simulink model "Registro_Harness2"  (R2020a)
settings: Solver=VariableStepAuto  StartTime=0.0  StopTime=10.0  RelTol=1e-3
settings Model: DataDictionary=Registro_variables.sldd  Creator=Juan  LastModifiedBy=Juan

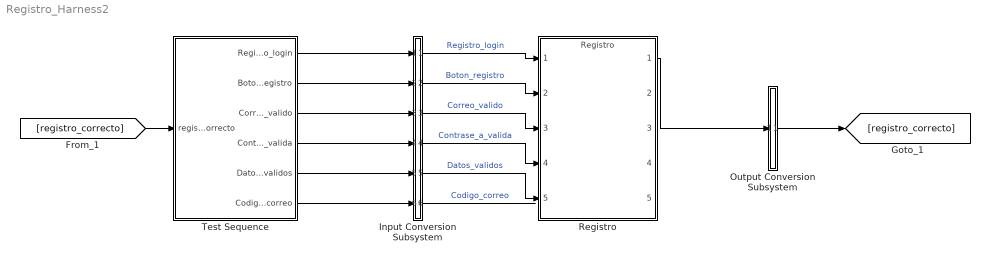
== system Registro_Harness2 ==
  Input Conversion Subsystem : Subsystem  Tag=__SLT_ICS__  Description=|
      | Signal spec.
      | and routing
      settings: AttributesFormatString=%<Description>
  Output Conversion Subsystem : Subsystem  Tag=__SLT_OCS__  Description=|
      | Signal spec.
      | and routing
      settings: AttributesFormatString=%<Description>
  Registro : ModelReference  ModelNameDialog=Registro  SimulationMode=Normal  ModelReferenceVersion=1.29
  Test Sequence : Test Sequence  TreatAsAtomicUnit=on
  wires:
  Test Sequence/1(Registro_login) -> Input Conversion Subsystem/1(Inport_1)
  Test Sequence/2(Boton_registro) -> Input Conversion Subsystem/2(Inport_2)
  Test Sequence/3(Correo_valido) -> Input Conversion Subsystem/3(Inport_3)
  Test Sequence/4(Contrase_a_valida) -> Input Conversion Subsystem/4(Inport_4)
  Test Sequence/5(Datos_validos) -> Input Conversion Subsystem/5(Inport_5)
  Test Sequence/6(Codigo_correo) -> Input Conversion Subsystem/6(Inport_6)
  [registro_correcto] -> Test Sequence/1(registro_correcto)
  Output Conversion Subsystem/1(Outport_1) -> [registro_correcto]
  Input Conversion Subsystem/1(Outport_1) -> Registro/1  "Registro_login"
  Input Conversion Subsystem/2(Outport_2) -> Registro/2  "Boton_registro"
  Input Conversion Subsystem/3(Outport_3) -> Registro/3  "Correo_valido"
  Input Conversion Subsystem/4(Outport_4) -> Registro/4  "Contrase_a_valida"
  Input Conversion Subsystem/5(Outport_5) -> Registro/5  "Datos_validos"
  Input Conversion Subsystem/6(Outport_6) -> ?  "Codigo_correo"
  Registro/1 -> Output Conversion Subsystem/1(Inport_1)

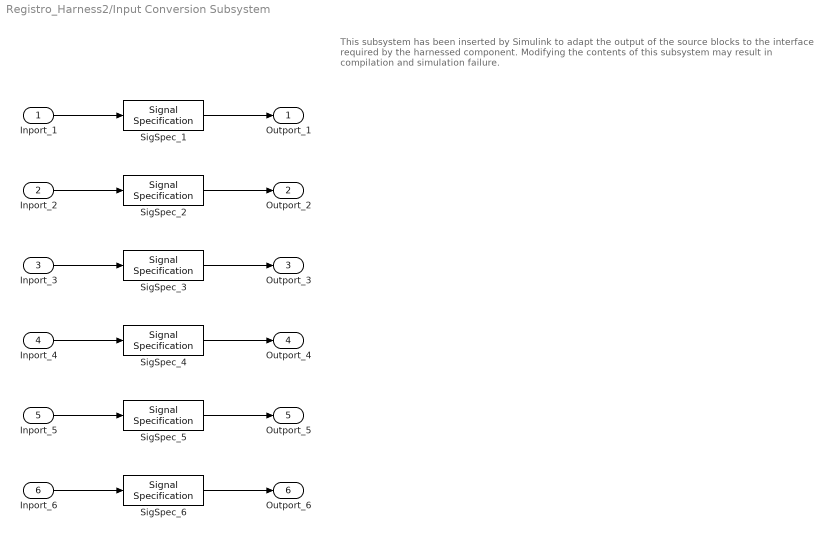
== system Registro_Harness2/Input Conversion Subsystem ==
  note: This subsystem has been inserted by Simulink to adapt the output of the source blocks to the interface required by the harnessed component.
      |  Modifying the contents of this subsystem may result in compilation and simulation failure.
  Inport_1 : Inport
  Inport_2 : Inport  Port=2
  Inport_3 : Inport  Port=3
  Inport_4 : Inport  Port=4
  Inport_5 : Inport  Port=5
  Inport_6 : Inport  Port=6
  SigSpec_1 : SignalSpecification  OutDataTypeStr=fixdt('int64')  Dimensions=[1]  SampleTime=[-1, 0]
  SigSpec_{2..6} (5 alike) : SignalSpecification  OutDataTypeStr=boolean  Dimensions=[1]  SampleTime=[-1, 0]
  Outport_1 : Outport
  Outport_2 : Outport  Port=2
  Outport_3 : Outport  Port=3
  Outport_4 : Outport  Port=4
  Outport_5 : Outport  Port=5
  Outport_6 : Outport  Port=6
  wires:
  SigSpec_1/1 -> Outport_1/1
  Inport_1/1 -> SigSpec_1/1
  SigSpec_2/1 -> Outport_2/1
  Inport_2/1 -> SigSpec_2/1
  SigSpec_3/1 -> Outport_3/1
  Inport_3/1 -> SigSpec_3/1
  SigSpec_4/1 -> Outport_4/1
  Inport_4/1 -> SigSpec_4/1
  SigSpec_5/1 -> Outport_5/1
  Inport_5/1 -> SigSpec_5/1
  SigSpec_6/1 -> Outport_6/1
  Inport_6/1 -> SigSpec_6/1

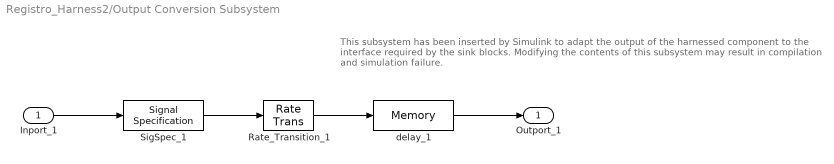
== system Registro_Harness2/Output Conversion Subsystem ==
  note: This subsystem has been inserted by Simulink to adapt the output of the harnessed component to the interface required by the sink blocks.
      |  Modifying the contents of this subsystem may result in compilation and simulation failure.
  Inport_1 : Inport
  Rate_Transition_1 : RateTransition  OutPortSampleTimeOpt=Inherit
  SigSpec_1 : SignalSpecification  OutDataTypeStr=boolean  Dimensions=[1]
  delay_1 : Memory
  Outport_1 : Outport
  wires:
  Inport_1/1 -> SigSpec_1/1
  SigSpec_1/1 -> Rate_Transition_1/1
  Rate_Transition_1/1 -> delay_1/1
  delay_1/1 -> Outport_1/1

== stateflow chart Registro_Harness2/Test Sequence ==
  settings: stateMachineType=SIMPLIFIED_MACHINE
  state Run
    %% Initialize data outputs.
    Registro_login(:) = 0; % fixed-point
    Boton_registro = false;
    Correo_valido = false;
    Contrase_a_valida = false;
    Datos_validos = false;
    Codigo_correo = false;
  (default) -> Run
  data: registro_correcto input boolean size=[1]; Registro_login output fixdt('int64') size=[1]; Boton_registro output boolean size=[1]; Correo_valido output boolean size=[1]; Contrase_a_valida output boolean size=[1]; Datos_validos output boolean size=[1]; Codigo_correo output boolean size=[1]
